simulink model "audio_loop_back"  (R2025b)
settings: Solver=VariableStepAuto  StartTime=0.0  StopTime=5  FixedStep=1024/48000  RelTol=1e-3
libraries: audiosources x1, dspsnks4 x1, dspsrcs4 x1
settings Model: Creator=saffeer  LastModifiedBy=saffeer
settings SolverCC: AllowMultiTaskInputOutput=on  ConcurrentTasks=on

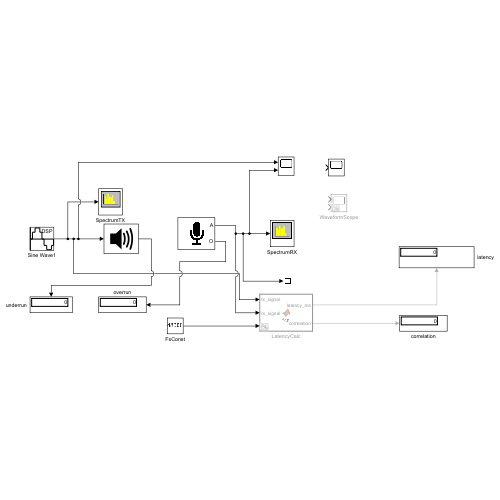
[thumbnail: Simulink's stored preview of the top-level diagram]
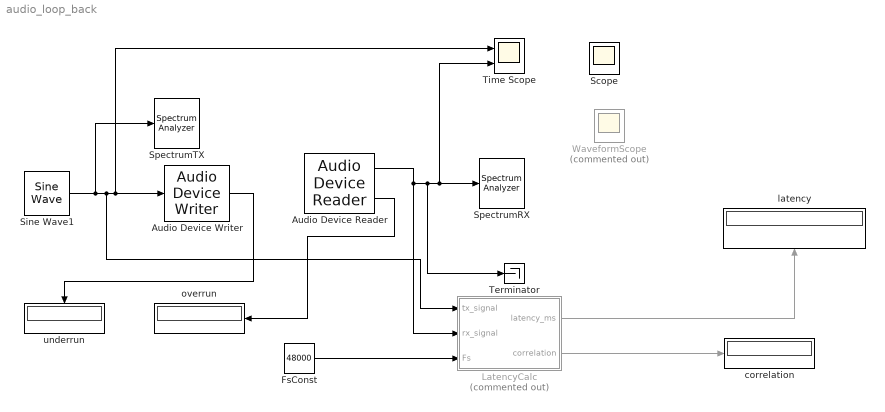
== system audio_loop_back ==
  Audio Device Reader : audiosources/Audio Device Reader  Driver=DirectSound  Device=Default  SampleRate=48000  NumChannels=2  SamplesPerFrame=1024  BitDepth=16-bit integer  NumBuffers=10  DefaultInputChannelMapping=on  InputChannelMapping=1:2  OutputNumOverrunSamples=on  OutputDataType=double  DriverIdx=1  DeviceWarnFlag=''
  Audio Device Writer : dspsnks4/Audio Device Writer  Driver=DirectSound  Device=Default  InheritSampleRate=on  SampleRate=44100  BitDepth=16-bit integer  BufferSize=4096  NumBuffers=10  DefaultOutputChannelMapping=on  OutputChannelMapping=1:2  OutputNumUnderrunSamples=on  DriverIdx=1  DeviceWarnFlag=''
  FsConst : Constant  Value=48000
  LatencyCalc : MATLAB Function  Commented=on  TreatAsAtomicUnit=on
  Scope : Scope
      settings: ActiveDisplayYMinimum=-1  ActiveDisplayYMaximum=1
  Sine Wave1 : dspsrcs4/Sine Wave  Amplitude=[0.2 0.4]  Frequency=[440 880]  Phase=0  SampleMode=Discrete  OutComplex=Real  CompMethod=Trigonometric fcn  TableSize=Speed  SampleTime=1/48000  SamplesPerFrame=1024  ResetState=Restart at time zero  OutputFrames=off  dataType=double  wordLen=16  udDataType=sfix(16)  fracBitsMode=Best precision  numFracBits=15  OutDataTypeStr=double  LastOutDataTypeStr=double
  SpectrumRX : SpectrumAnalyzer  WindowPosition=[0.000000,36.000000,1280.000000,649.000000,]  Visible=on  ScopeFrameLocation=window  SpectrumType=Power density  ViewType=Spectrum and spectrogram  SampleRateSource=Property  SampleRate=48000  PlotAsTwoSidedSpectrum=off  WindowInvariantSamplesPerUpdate=on  Span=24000  CenterFrequency=12000  StartFrequency=0  StopFrequency=24000  SpectrumUnits=dBm/Hz  TimeSpan=1  YLimits=[-121.0408 15.6059]  ColorLimits=[-121.0408 15.6059]  SelectedToolstripTab=spectrumAnalyzerToolstrip.spectrogramTab
  SpectrumTX : SpectrumAnalyzer  WindowPosition=[703.000000,80.000000,565.000000,529.000000,]  Visible=on  ScopeFrameLocation=window  SpectrumType=Power density  ViewType=Spectrum and spectrogram  SampleRateSource=Property  SampleRate=48000  PlotAsTwoSidedSpectrum=off  WindowInvariantSamplesPerUpdate=on  Span=24000  CenterFrequency=12000  StartFrequency=0  StopFrequency=24000  SpectrumUnits=dBm/Hz  YLimits=[-134.7313 17.1291]  ColorLimits=[-134.7313 17.1291]  SelectedToolstripTab=spectrumAnalyzerToolstrip.channelMeasurementsTab
  Terminator : Terminator
  Time Scope : Scope  NumInputPorts=2
      settings: TimeUnits=Metric (based on Time Span)  ActiveDisplayYMinimum=-0.23466701382861777  ActiveDisplayYMaximum=0.24152346236185848  YLabel=Amplitude  DataLoggingVariableName=ScopeData2
  WaveformScope : Scope  Commented=on  NumInputPorts=2
      settings: ActiveDisplayYMinimum=-1  ActiveDisplayYMaximum=1
  correlation : Display
  latency : Display
  overrun : Display
  underrun : Display
  wires:
  Sine Wave1/1 -> SpectrumTX/1, LatencyCalc/1(tx_signal), Time Scope/1, Audio Device Writer/1
  Audio Device Reader/1 -> LatencyCalc/2(rx_signal), Terminator/1, Time Scope/2, SpectrumRX/1
  FsConst/1 -> LatencyCalc/3(Fs)
  LatencyCalc/1(latency_ms) -> latency/1
  LatencyCalc/2(correlation) -> correlation/1
  Audio Device Writer/1 -> underrun/1
  Audio Device Reader/2 -> overrun/1

== matlab function audio_loop_back/LatencyCalc ==
  data: tx_signal input; latency_ms output; rx_signal input; Fs input; correlation output
function [latency_ms, correlation] = fcn(tx_signal, rx_signal, Fs)
%#codegen
% Latency Calculator using Cross-Correlation
%
% This function measures the round-trip latency between transmitted and
% received audio signals using cross-correlation.
%
% Inputs:
%   tx_signal   - Transmitted signal frame (column vector)
%   rx_signal   - Received signal frame (column vector)
%   Fs          - Sample rate in Hz
%
% Outputs:
%   latency_ms  - Measured latency in milliseconds
%   correlation - Normalized correlation coefficient (0-1)


persistent buffer_tx buffer_rx
bufferSize = 4096;  % Buffer size for correlation (adjust if needed)
frameSize = length(tx_signal);

% Initialize buffers on first call
if isempty(buffer_tx)
    buffer_tx = zeros(bufferSize, 1);
    buffer_rx = zeros(bufferSize, 1);
end

% Update circular buffers with new frame data
buffer_tx = [buffer_tx(frameSize+1:end); tx_signal(:)];
buffer_rx = [buffer_rx(frameSize+1:end); rx_signal(:)];

% Cross-correlation to find delay
maxLag = bufferSize/2;
[xcorr_result, lags] = xcorr(buffer_rx, buffer_tx, maxLag);

% Find peak correlation
[maxVal, maxIdx] = max(abs(xcorr_result));
delay_samples = lags(maxIdx);

% Convert delay to milliseconds
latency_ms = double(delay_samples) / double(Fs) * 1000;

% Calculate normalized correlation coefficient
norm_tx = sqrt(sum(buffer_tx.^2));
norm_rx = sqrt(sum(buffer_rx.^2));
correlation = maxVal / (norm_tx * norm_rx + 1e-10);

end
